simulink model "Exemplo3"  (R2021a)
settings: Solver=VariableStepAuto  StartTime=0.0  StopTime=10.0  MaxStep=100  RelTol=1e-3
settings Model: Creator=taffarel55  LastModifiedBy=taffarel55

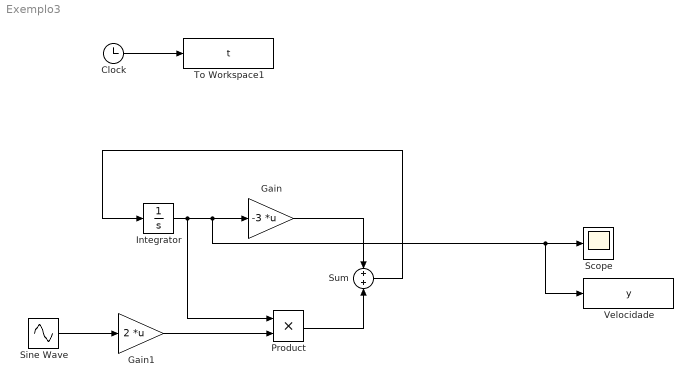
== system Exemplo3 ==
  Clock : Clock
  Gain : Gain  Gain=-3  Multiplication=Matrix(K*u)
  Gain1 : Gain  Gain=2  Multiplication=Matrix(K*u)
  Integrator : Integrator  InitialCondition=1
  Product : Product
  Scope : Scope
  Sine Wave : Sin  SampleTime=0
  Sum : Sum
  To Workspace1 : ToWorkspace  VariableName=t  SaveFormat=Timeseries  SampleTime=-1
  Velocidade : ToWorkspace  VariableName=y  SampleTime=-1
  wires:
  Clock/1 -> To Workspace1/1
  Gain/1 -> Sum/1
  Integrator/1 -> Product/1, Velocidade/1, Scope/1, Gain/1
  Product/1 -> Sum/2
  Sine Wave/1 -> Gain1/1
  Gain1/1 -> Product/2
  Sum/1 -> Integrator/1
